simulink model "mfilt_cicdecimzerolat"  (Simulink 5.0)
settings: Solver=ode45  StartTime=0.0  StopTime=10.0  RelTol=1e-3
values from neighbouring files (symbols this model uses):
  R = 64    [firceqripdemo.m]    (also in firgrdemo.m = [0.1]; firnyquistdemo.m = 0.5; firtransdemo.m = [0.1 0.05]; ifirdemo.m = [Rpass Rstop])
libraries: dspobslib x4, dspsigops x1
settings Model: Creator=pc  LastModifiedBy=pc  BooleanDataType=off

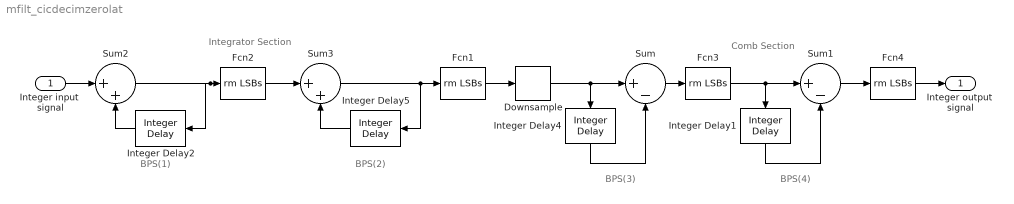
== system mfilt_cicdecimzerolat ==
  note: Integrator Section
  note: Comb Section
  note: BPS(1)
  note: BPS(2)
  note: BPS(3)
  note: BPS(4)
  Integer input  signal : Inport
  Downsample : dspsigops/Downsample  N=R  phase=0  ic=0  smode=Allow multirate  fmode=Maintain input frame size
  Fcn{1..4} (4 alike) : Fcn  Expr=rm LSBs
  Integer Delay1 : dspobslib/Integer Delay  Orientation=down  delay=M  ic=0  reset_popup=None
  Integer Delay2 : dspobslib/Integer Delay  Orientation=left  delay=1  ic=0  reset_popup=None
  Integer Delay4 : dspobslib/Integer Delay  Orientation=down  delay=M  ic=0  reset_popup=None
  Integer Delay5 : dspobslib/Integer Delay  Orientation=left  delay=1  ic=0  reset_popup=None
  Sum : Sum  Inputs=|+-  SaturateOnIntegerOverflow=on  InputSameDT=on
  Sum1 : Sum  Inputs=|+-  SaturateOnIntegerOverflow=on  InputSameDT=on
  Sum2 : Sum  Inputs=|++  SaturateOnIntegerOverflow=on  InputSameDT=on
  Sum3 : Sum  Inputs=|++  SaturateOnIntegerOverflow=on  InputSameDT=on
  Integer output  signal : Outport
  wires:
  Integer Delay4/1 -> Sum/2
  Sum/1 -> Fcn3/1
  Downsample/1 -> Sum/1, Integer Delay4/1
  Sum2/1 -> Fcn2/1, Integer Delay2/1
  Fcn1/1 -> Downsample/1
  Fcn2/1 -> Sum3/1
  Integer Delay1/1 -> Sum1/2
  Sum1/1 -> Fcn4/1
  Fcn3/1 -> Sum1/1, Integer Delay1/1
  Sum3/1 -> Fcn1/1, Integer Delay5/1
  Integer input  signal/1 -> Sum2/1
  Fcn4/1 -> Integer output  signal/1
  Integer Delay2/1 -> Sum2/2
  Integer Delay5/1 -> Sum3/2
